simulink model "modelos_equivalentes_para_informe"  (R2019a)
settings: Solver=VariableStepAuto  StartTime=0.0  StopTime=10.0  RelTol=1e-3
undefined symbols (not defined in the file): K_d, K_i, K_p
libraries: simulink x1
settings Model: Creator=pedro  LastModifiedBy=pedro

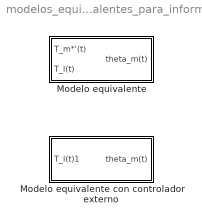
== system modelos_equivalentes_para_informe ==
  Modelo equivalente : Subsystem
  Modelo equivalente con controlador externo : Subsystem

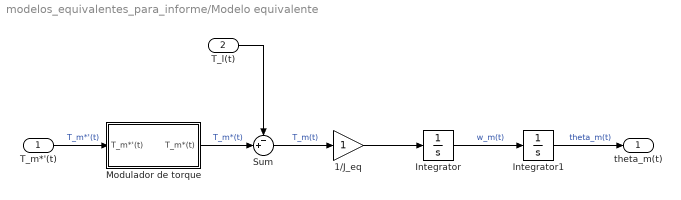
== system modelos_equivalentes_para_informe/Modelo equivalente ==
  T_m*'(t) : Inport
  T_l(t) : Inport  Port=2
  1/J_eq : Gain
  Integrator : Integrator
  Integrator1 : Integrator
  Modulador de torque : Subsystem
  Sum : Sum  Inputs=-+|
  theta_m(t) : Outport
  wires:
  Sum/1 -> 1/J_eq/1  "T_m(t)"
  Integrator/1 -> Integrator1/1  "w_m(t)"
  Integrator1/1 -> theta_m(t)/1  "theta_m(t)"
  T_m*'(t)/1 -> Modulador de torque/1(T_m*'(t))  "T_m*'(t)"
  1/J_eq/1 -> Integrator/1
  T_l(t)/1 -> Sum/1
  Modulador de torque/1(T_m*(t)) -> Sum/2  "T_m*(t)"

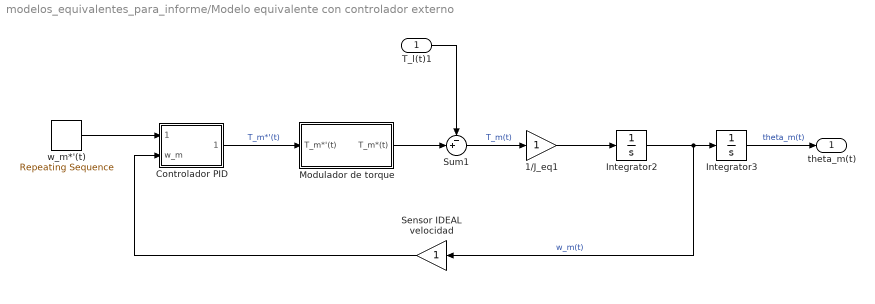
== system modelos_equivalentes_para_informe/Modelo equivalente con controlador externo ==
  T_l(t)1 : Inport
  1/J_eq1 : Gain
  Controlador PID : Subsystem
  Integrator2 : Integrator
  Integrator3 : Integrator
  Modulador de torque : Subsystem
  Sensor IDEAL velocidad : Gain
  Sum1 : Sum  Inputs=-+|
  w_m*'(t) : simulink/Sources/Repeating Sequence  rep_seq_t=[0 0.099 0.1 0.699 0.7 10]  rep_seq_y=[0 0 420 420 0 0]
  theta_m(t) : Outport
  wires:
  Sensor IDEAL velocidad/1 -> Controlador PID/2(w_m)
  Integrator3/1 -> theta_m(t)/1  "theta_m(t)"
  Integrator2/1 -> Sensor IDEAL velocidad/1, Integrator3/1  "w_m(t)"
  1/J_eq1/1 -> Integrator2/1
  T_l(t)1/1 -> Sum1/1
  Controlador PID/1(T_m*'(t)) -> Modulador de torque/1(T_m*'(t))  "T_m*'(t)"
  Modulador de torque/1(T_m*(t)) -> Sum1/2
  Sum1/1 -> 1/J_eq1/1  "T_m(t)"
  w_m*'(t)/1 -> Controlador PID/1(w_m*)

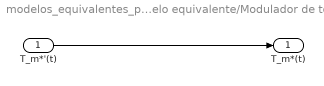
== system modelos_equivalentes_para_informe/Modelo equivalente/Modulador de torque ==
  T_m*'(t) : Inport
  T_m*(t) : Outport
  wires:
  T_m*'(t)/1 -> T_m*(t)/1

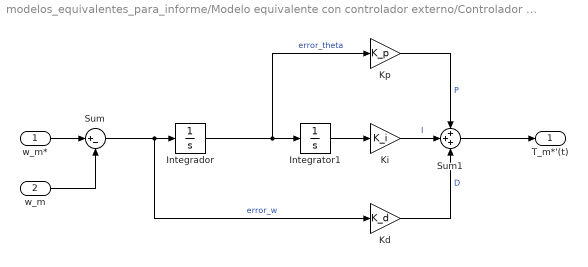
== system modelos_equivalentes_para_informe/Modelo equivalente con controlador externo/Controlador PID ==
  w_m* : Inport
  w_m : Inport  Port=2
  Integrador : Integrator
  Integrator1 : Integrator
  Kd : Gain  Gain=K_d
  Ki : Gain  Gain=K_i
  Kp : Gain  Gain=K_p
  Sum : Sum  Inputs=|+-
  Sum1 : Sum  Inputs=+++
  T_m*'(t) : Outport
  wires:
  Sum/1 -> Kd/1, Integrador/1  "error_w"
  w_m/1 -> Sum/2
  Sum1/1 -> T_m*'(t)/1
  Integrador/1 -> Integrator1/1, Kp/1  "error_theta"
  Kd/1 -> Sum1/3  "D"
  Integrator1/1 -> Ki/1
  w_m*/1 -> Sum/1
  Ki/1 -> Sum1/2  "I"
  Kp/1 -> Sum1/1  "P"

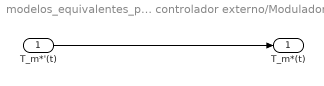
== system modelos_equivalentes_para_informe/Modelo equivalente con controlador externo/Modulador de torque ==
  T_m*'(t) : Inport
  T_m*(t) : Outport
  wires:
  T_m*'(t)/1 -> T_m*(t)/1
